simulink model "hcci_eng"  (R2018a)
settings: Solver=VariableStepAuto  StartTime=0.0  StopTime=t_end  RelTol=1e-3
values from neighbouring files (symbols this model uses):
  A01 = f(90)    [load_param.m]
  A2 = 0.3149    [load_param.m]
  A20 = f(70)    [load_param.m]
  alpha = 0.5794    [load_param.m]
  beta_0 = 1.035    [load_param.m]
  beta_1 = 1.1568    [load_param.m]
  gamma = 1.4    [load_param.m]
  h2 = 267    [load_param.m]
  kappa_0 = 0.5729    [load_param.m]
  kappa_1 = -0.52039    [load_param.m]
  m1_0 = states(end,1)    [hcci_sim.m]
  m2_0 = states(end,3)    [hcci_sim.m]
  p0 = 101000    [load_param.m]
  p2_0 = states(end,2)    [hcci_sim.m]
  R = 296.25    [HCCI_Combustion.m]    (also in load_param.m)
  T1 = 90 + 273.15    (= 363.15)    [load_param.m]
  T_w = 400    [load_param.m]
  tau = 120/N    (= 0.12)    [Validation.m]    (also in load_param.m)
  u_rbl = 3    [load_param.m]
  V1 = 0.0013    [load_param.m]
  V2 = 0.015    [load_param.m]
  V_BDC = V_ivc    (= 0.000592307692308)    [load_param.m]
  V_ivc = double(subs(Vc, theta, theta_ivc))    [HCCI_Combustion.m]    (also in load_param.m = 0.000592307692308)
  Wf = 11.9e-6    (= 1.19e-05)    [load_param.m]
undefined symbols (not defined in the file or in its folder): C_d
settings Model: Creator=Lenovo  LastModifiedBy=Lenovo

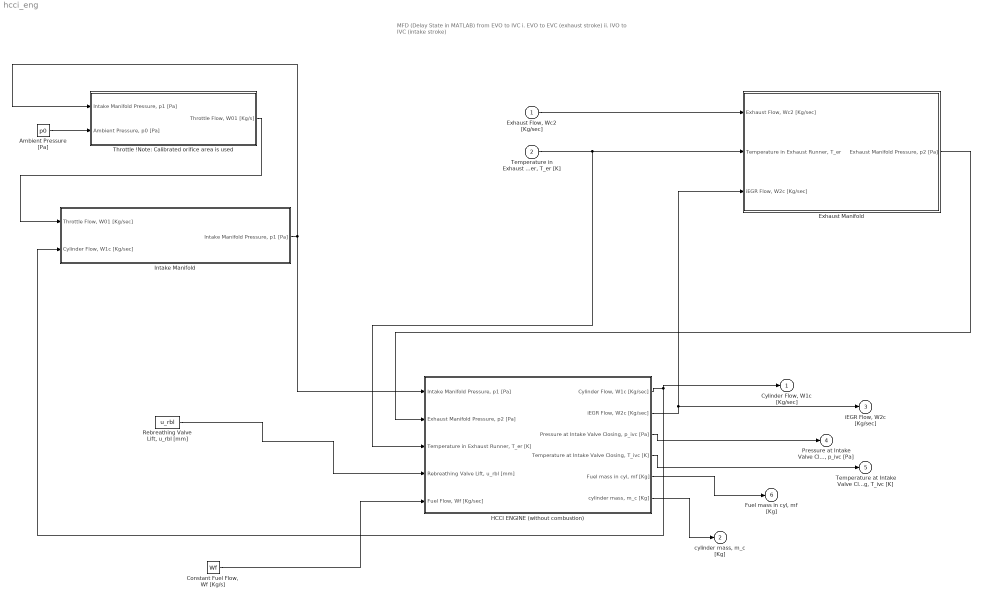
== system hcci_eng ==
  note: MFD (Delay State in MATLAB) from EVO to IVC
      | i. EVO to EVC (exhaust stroke)
      | ii. IVO to IVC (intake stroke)
  "Exhaust Flow, Wc2 [Kg/sec]" : Inport
  "Temperature in Exhaust Runner, T_er [K]" : Inport  Port=2
  Ambient Pressure [Pa] : Constant  Value=p0
  "Constant Fuel Flow, Wf [Kg/s] " : Constant  Value=Wf
  Exhaust Manifold : Subsystem
  HCCI ENGINE (without combustion) : Subsystem
  Intake Manifold : Subsystem
  "Rebreathing Valve Lift, u_rbl [mm]" : Constant  Value=u_rbl
  Throttle !Note: Calibrated orifice area is used : Subsystem
  "Cylinder Flow, W1c [Kg/sec]" : Outport
  "cylinder mass, m_c [Kg]" : Outport  Port=2
  "iEGR Flow, W2c [Kg/sec]" : Outport  Port=3
  "Pressure at Intake Valve Closing, p_ivc [Pa]" : Outport  Port=4
  "Temperature at Intake Valve Closing, T_ivc [K]" : Outport  Port=5
  "Fuel mass in cyl, mf [Kg]" : Outport  Port=6
  wires:
  Ambient Pressure [Pa]/1 -> Throttle !Note: Calibrated orifice area is used/2("Ambient Pressure, p0 [Pa]")
  Throttle !Note: Calibrated orifice area is used/1("Throttle Flow, W01 [Kg/s]") -> Intake Manifold/1("Throttle Flow, W01 [Kg/sec]")
  Intake Manifold/1("Intake Manifold Pressure, p1 [Pa]") -> HCCI ENGINE (without combustion)/1("Intake Manifold Pressure, p1 [Pa]"), Throttle !Note: Calibrated orifice area is used/1("Intake Manifold Pressure, p1 [Pa]")
  HCCI ENGINE (without combustion)/2("iEGR Flow, W2c [Kg/sec]") -> Exhaust Manifold/3("iEGR Flow, W2c [Kg/sec]"), "iEGR Flow, W2c [Kg/sec]"/1
  "Exhaust Flow, Wc2 [Kg/sec]"/1 -> Exhaust Manifold/1("Exhaust Flow, Wc2 [Kg/sec]")
  "Temperature in Exhaust Runner, T_er [K]"/1 -> Exhaust Manifold/2("Temperature in Exhaust Runner, T_er"), HCCI ENGINE (without combustion)/3("Temperature in Exhaust Runner, T_er [K]")
  Exhaust Manifold/1("Exhaust Manifold Pressure, p2 [Pa]") -> HCCI ENGINE (without combustion)/2("Exhaust Manifold Pressure, p2 [Pa]")
  "Constant Fuel Flow, Wf [Kg/s] "/1 -> HCCI ENGINE (without combustion)/5("Fuel Flow, Wf [Kg/sec] ")
  "Rebreathing Valve Lift, u_rbl [mm]"/1 -> HCCI ENGINE (without combustion)/4("Rebreathing Valve Lift, u_rbl [mm]")
  HCCI ENGINE (without combustion)/1("Cylinder Flow, W1c [Kg/sec]") -> "Cylinder Flow, W1c [Kg/sec]"/1, Intake Manifold/2("Cylinder Flow, W1c [Kg/sec]")
  HCCI ENGINE (without combustion)/3("Pressure at Intake Valve Closing, p_ivc [Pa]") -> "Pressure at Intake Valve Closing, p_ivc [Pa]"/1
  HCCI ENGINE (without combustion)/4("Temperature at Intake Valve Closing, T_ivc [K]") -> "Temperature at Intake Valve Closing, T_ivc [K]"/1
  HCCI ENGINE (without combustion)/5("Fuel mass in cyl, mf [Kg]") -> "Fuel mass in cyl, mf [Kg]"/1
  HCCI ENGINE (without combustion)/6("cylinder mass, m_c [Kg]") -> "cylinder mass, m_c [Kg]"/1

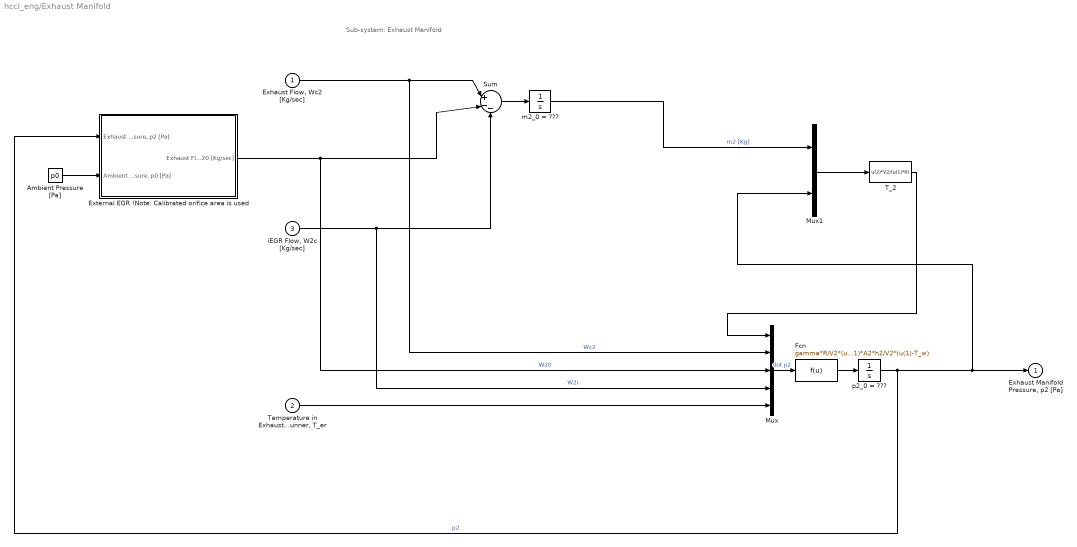
== system hcci_eng/Exhaust Manifold ==
  note: Sub-system: Exhaust Manifold
  "Exhaust Flow, Wc2 [Kg/sec]" : Inport
  "Temperature in Exhaust Runner, T_er" : Inport  Port=2
  "iEGR Flow, W2c [Kg/sec]" : Inport  Port=3
  Ambient Pressure [Pa] : Constant  Value=p0
  "External EGR !Note: Calibrated orifice area is used " : Subsystem
  Fcn : Fcn  Expr=gamma*R/V2*(u(2)*u(5)-(u(3)+u(4))*u(1))-(gamma-1)*A2*h2/V2*(u(1)-T_w)
  Mux : Mux  Inputs=5
  Mux1 : Mux  Inputs=2
  Sum : Sum  Inputs=|+--
  T_2 : Fcn  Expr=u(2)*V2/(u(1)*R)
  m2_0 = ??? : Integrator  InitialCondition=m2_0
  p2_0 = ??? : Integrator  InitialCondition=p2_0
  "Exhaust Manifold Pressure, p2 [Pa]" : Outport
  wires:
  "Exhaust Flow, Wc2 [Kg/sec]"/1 -> Mux/2, Sum/1  "Wc2"
  "External EGR !Note: Calibrated orifice area is used "/1("Exhaust Flow, W20 [Kg/sec]") -> Mux/3, Sum/2  "W20"
  "iEGR Flow, W2c [Kg/sec]"/1 -> Mux/4, Sum/3  "W2c"
  Sum/1 -> m2_0 = ???/1
  p2_0 = ???/1 -> Mux1/2, "Exhaust Manifold Pressure, p2 [Pa]"/1, "External EGR !Note: Calibrated orifice area is used "/1("Exhaust Manifold Pressure, p2 [Pa]")  "p2"
  Ambient Pressure [Pa]/1 -> "External EGR !Note: Calibrated orifice area is used "/2("Ambient Pressure, p0 [Pa]")
  "Temperature in Exhaust Runner, T_er"/1 -> Mux/5
  T_2/1 -> Mux/1
  Mux/1 -> Fcn/1  "dot p2"
  Fcn/1 -> p2_0 = ???/1
  Mux1/1 -> T_2/1
  m2_0 = ???/1 -> Mux1/1  "m2 [Kg]"

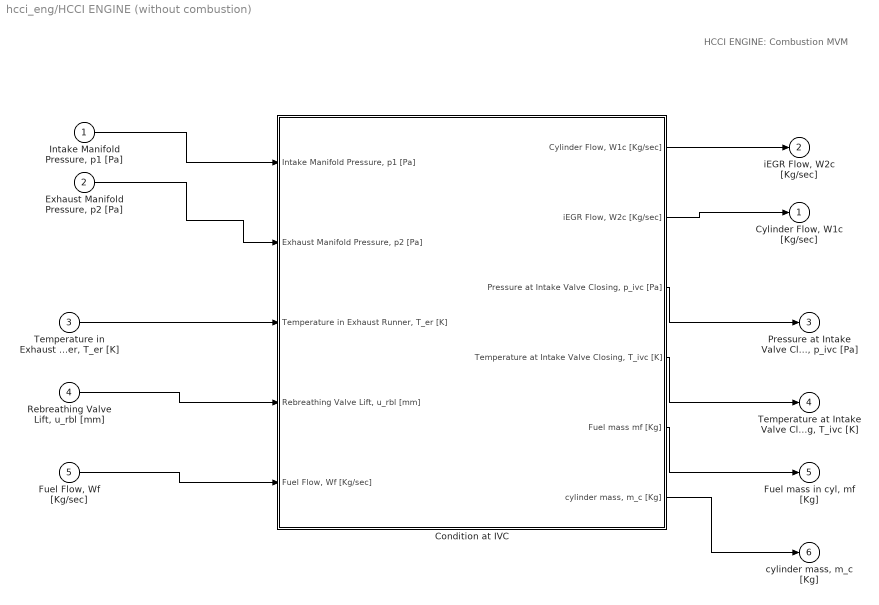
== system hcci_eng/HCCI ENGINE (without combustion) ==
  note: HCCI ENGINE: Combustion MVM
  "Intake Manifold Pressure, p1 [Pa]" : Inport
  "Exhaust Manifold Pressure, p2 [Pa]" : Inport  Port=2
  "Temperature in Exhaust Runner, T_er [K]" : Inport  Port=3
  "Rebreathing Valve Lift, u_rbl [mm]" : Inport  Port=4
  "Fuel Flow, Wf [Kg/sec] " : Inport  Port=5
  Condition at IVC : Subsystem
  "Cylinder Flow, W1c [Kg/sec]" : Outport
  "iEGR Flow, W2c [Kg/sec]" : Outport  Port=2
  "Pressure at Intake Valve Closing, p_ivc [Pa]" : Outport  Port=3
  "Temperature at Intake Valve Closing, T_ivc [K]" : Outport  Port=4
  "Fuel mass in cyl, mf [Kg]" : Outport  Port=5
  "cylinder mass, m_c [Kg]" : Outport  Port=6
  wires:
  "Intake Manifold Pressure, p1 [Pa]"/1 -> Condition at IVC/1("Intake Manifold Pressure, p1 [Pa]")
  "Exhaust Manifold Pressure, p2 [Pa]"/1 -> Condition at IVC/2("Exhaust Manifold Pressure, p2 [Pa]")
  "Temperature in Exhaust Runner, T_er [K]"/1 -> Condition at IVC/3("Temperature in Exhaust Runner, T_er [K]")
  "Rebreathing Valve Lift, u_rbl [mm]"/1 -> Condition at IVC/4("Rebreathing Valve Lift, u_rbl [mm]")
  "Fuel Flow, Wf [Kg/sec] "/1 -> Condition at IVC/5("Fuel Flow, Wf [Kg/sec] ")
  Condition at IVC/1("Cylinder Flow, W1c [Kg/sec]") -> "iEGR Flow, W2c [Kg/sec]"/1
  Condition at IVC/2("iEGR Flow, W2c [Kg/sec]") -> "Cylinder Flow, W1c [Kg/sec]"/1
  Condition at IVC/3("Pressure at Intake Valve Closing, p_ivc [Pa]") -> "Pressure at Intake Valve Closing, p_ivc [Pa]"/1
  Condition at IVC/4("Temperature at Intake Valve Closing, T_ivc [K]") -> "Temperature at Intake Valve Closing, T_ivc [K]"/1
  Condition at IVC/5(Fuel mass mf [Kg]) -> "Fuel mass in cyl, mf [Kg]"/1
  Condition at IVC/6("cylinder mass, m_c [Kg]") -> "cylinder mass, m_c [Kg]"/1

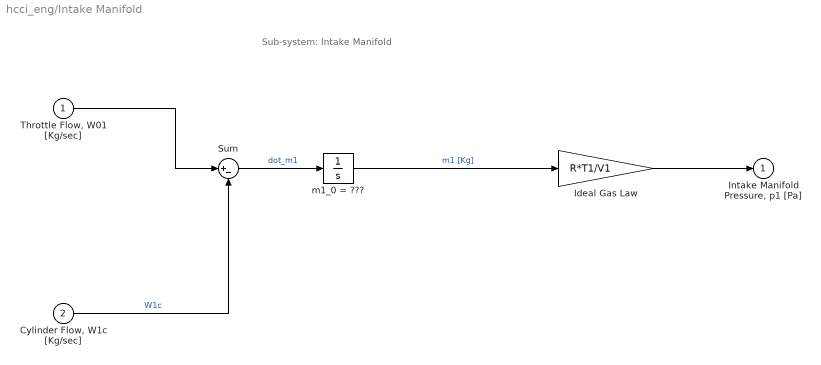
== system hcci_eng/Intake Manifold ==
  note: Sub-system: Intake Manifold
  "Throttle Flow, W01 [Kg/sec]" : Inport
  "Cylinder Flow, W1c [Kg/sec]" : Inport  Port=2
  Ideal Gas Law : Gain  Gain=R*T1/V1
  Sum : Sum  Inputs=|+-
  m1_0 = ??? : Integrator  InitialCondition=m1_0
  "Intake Manifold Pressure, p1 [Pa]" : Outport
  wires:
  "Cylinder Flow, W1c [Kg/sec]"/1 -> Sum/2  "W1c"
  "Throttle Flow, W01 [Kg/sec]"/1 -> Sum/1
  Sum/1 -> m1_0 = ???/1  "dot_m1"
  m1_0 = ???/1 -> Ideal Gas Law/1  "m1 [Kg]"
  Ideal Gas Law/1 -> "Intake Manifold Pressure, p1 [Pa]"/1

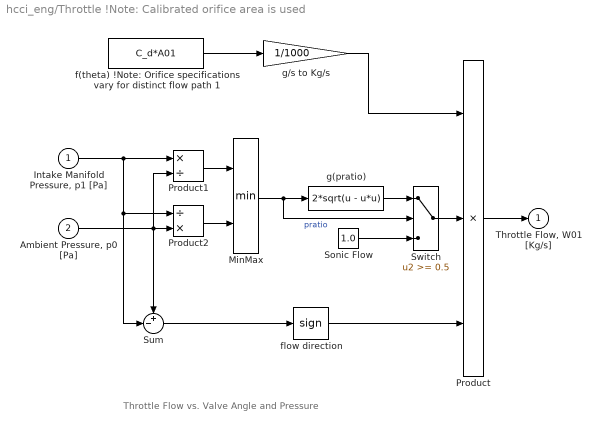
== system hcci_eng/Throttle !Note: Calibrated orifice area is used ==
  note: Throttle Flow vs. Valve Angle and Pressure
  "Intake Manifold Pressure, p1 [Pa]" : Inport
  "Ambient Pressure, p0 [Pa]" : Inport  Port=2
  MinMax : MinMax  Inputs=2  SaturateOnIntegerOverflow=on  InputSameDT=on
  Product : Product  Inputs=3  SaturateOnIntegerOverflow=on  RndMeth=Zero  InputSameDT=on  OutDataTypeStr=Inherit: Same as first input
  Product1 : Product  Inputs=*/  SaturateOnIntegerOverflow=on  RndMeth=Zero  InputSameDT=on  OutDataTypeStr=Inherit: Same as first input
  Product2 : Product  Inputs=/*  SaturateOnIntegerOverflow=on  RndMeth=Zero  InputSameDT=on  OutDataTypeStr=Inherit: Same as first input
  "Sonic Flow " : Constant  Value=1.0
  Sum : Sum  Inputs=+-|  SaturateOnIntegerOverflow=on  InputSameDT=on  OutDataTypeStr=Inherit: Same as first input
  Switch : Switch  Threshold=0.5  SaturateOnIntegerOverflow=on  InputSameDT=on
  f(theta) !Note: Orifice specifications vary for distinct flow path 1 : Constant  Value=C_d*A01
  flow direction : Signum
  g(pratio) : Fcn  Expr=2*sqrt(u - u*u)
  g/s to Kg/s : Gain  Gain=1/1000
  "Throttle Flow, W01 [Kg/s]" : Outport  InitialOutput=0
  wires:
  "Intake Manifold Pressure, p1 [Pa]"/1 -> Sum/2, Product2/1, Product1/1
  Product2/1 -> MinMax/2
  Product1/1 -> MinMax/1
  "Ambient Pressure, p0 [Pa]"/1 -> Sum/1, Product2/2, Product1/2
  g(pratio)/1 -> Switch/1
  "Sonic Flow "/1 -> Switch/3
  Switch/1 -> Product/2
  flow direction/1 -> Product/3
  Sum/1 -> flow direction/1
  MinMax/1 -> Switch/2, g(pratio)/1  "pratio"
  Product/1 -> "Throttle Flow, W01 [Kg/s]"/1
  f(theta) !Note: Orifice specifications vary for distinct flow path 1/1 -> g/s to Kg/s/1
  g/s to Kg/s/1 -> Product/1

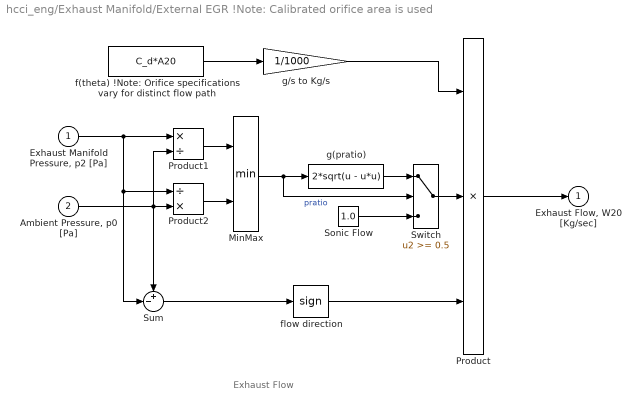
== system hcci_eng/Exhaust Manifold/External EGR !Note: Calibrated orifice area is used  ==
  note: Exhaust Flow
  "Exhaust Manifold Pressure, p2 [Pa]" : Inport
  "Ambient Pressure, p0 [Pa]" : Inport  Port=2
  MinMax : MinMax  Inputs=2  SaturateOnIntegerOverflow=on  InputSameDT=on
  Product : Product  Inputs=3  SaturateOnIntegerOverflow=on  RndMeth=Zero  InputSameDT=on  OutDataTypeStr=Inherit: Same as first input
  Product1 : Product  Inputs=*/  SaturateOnIntegerOverflow=on  RndMeth=Zero  InputSameDT=on  OutDataTypeStr=Inherit: Same as first input
  Product2 : Product  Inputs=/*  SaturateOnIntegerOverflow=on  RndMeth=Zero  InputSameDT=on  OutDataTypeStr=Inherit: Same as first input
  "Sonic Flow " : Constant  Value=1.0
  Sum : Sum  Inputs=+-|  SaturateOnIntegerOverflow=on  InputSameDT=on  OutDataTypeStr=Inherit: Same as first input
  Switch : Switch  Threshold=0.5  SaturateOnIntegerOverflow=on  InputSameDT=on
  "f(theta) !Note: Orifice specifications vary for distinct flow path " : Constant  Value=C_d*A20
  flow direction : Signum
  g(pratio) : Fcn  Expr=2*sqrt(u - u*u)
  g/s to Kg/s : Gain  Gain=1/1000
  "Exhaust Flow, W20 [Kg/sec]" : Outport  InitialOutput=0
  wires:
  "Exhaust Manifold Pressure, p2 [Pa]"/1 -> Sum/2, Product2/1, Product1/1
  Product2/1 -> MinMax/2
  Product1/1 -> MinMax/1
  "Ambient Pressure, p0 [Pa]"/1 -> Sum/1, Product2/2, Product1/2
  g(pratio)/1 -> Switch/1
  "Sonic Flow "/1 -> Switch/3
  Switch/1 -> Product/2
  flow direction/1 -> Product/3
  Sum/1 -> flow direction/1
  MinMax/1 -> Switch/2, g(pratio)/1  "pratio"
  Product/1 -> "Exhaust Flow, W20 [Kg/sec]"/1
  "f(theta) !Note: Orifice specifications vary for distinct flow path "/1 -> g/s to Kg/s/1
  g/s to Kg/s/1 -> Product/1

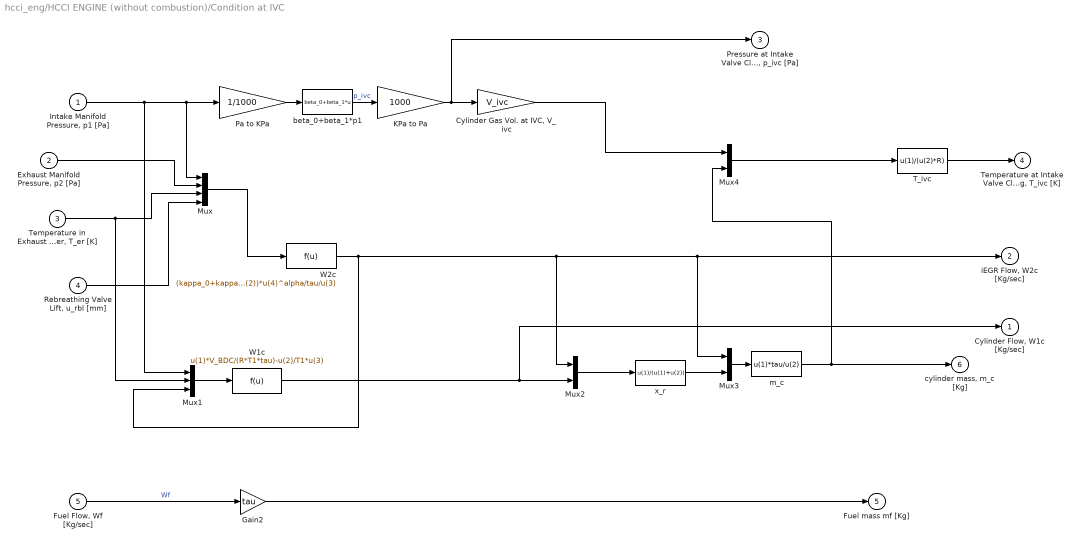
== system hcci_eng/HCCI ENGINE (without combustion)/Condition at IVC ==
  "Intake Manifold Pressure, p1 [Pa]" : Inport
  "Exhaust Manifold Pressure, p2 [Pa]" : Inport  Port=2
  "Temperature in Exhaust Runner, T_er [K]" : Inport  Port=3
  "Rebreathing Valve Lift, u_rbl [mm]" : Inport  Port=4
  "Fuel Flow, Wf [Kg/sec] " : Inport  Port=5
  "Cylinder Gas Vol. at IVC, V_ivc" : Gain  Gain=V_ivc
  Gain2 : Gain  Gain=tau
  KPa to Pa : Gain  Gain=1000
  Mux : Mux
  Mux1 : Mux  Inputs=3
  Mux2 : Mux  Inputs=2
  Mux3 : Mux  Inputs=2
  Mux4 : Mux  Inputs=2
  Pa to KPa : Gain  Gain=1/1000
  T_ivc : Fcn  Expr=u(1)/(u(2)*R)
  W1c : Fcn  Expr=u(1)*V_BDC/(R*T1*tau)-u(2)/T1*u(3)
  W2c : Fcn  Expr=(kappa_0+kappa_1*u(1)/u(2))*u(4)^alpha/tau/u(3)
  beta_0+beta_1*p1 : Fcn  Expr=beta_0+beta_1*u
  m_c : Fcn  Expr=u(1)*tau/u(2)
  x_r : Fcn  Expr=u(1)/(u(1)+u(2))
  "Cylinder Flow, W1c [Kg/sec]" : Outport
  "iEGR Flow, W2c [Kg/sec]" : Outport  Port=2
  "Pressure at Intake Valve Closing, p_ivc [Pa]" : Outport  Port=3
  "Temperature at Intake Valve Closing, T_ivc [K]" : Outport  Port=4
  Fuel mass mf [Kg] : Outport  Port=5
  "cylinder mass, m_c [Kg]" : Outport  Port=6
  wires:
  beta_0+beta_1*p1/1 -> KPa to Pa/1  "p_ivc"
  Mux/1 -> W2c/1
  "Temperature in Exhaust Runner, T_er [K]"/1 -> Mux1/2, Mux/3
  "Rebreathing Valve Lift, u_rbl [mm]"/1 -> Mux/4
  "Fuel Flow, Wf [Kg/sec] "/1 -> Gain2/1  "Wf"
  "Intake Manifold Pressure, p1 [Pa]"/1 -> Mux1/1, Mux/1, Pa to KPa/1
  "Exhaust Manifold Pressure, p2 [Pa]"/1 -> Mux/2
  Pa to KPa/1 -> beta_0+beta_1*p1/1
  KPa to Pa/1 -> "Pressure at Intake Valve Closing, p_ivc [Pa]"/1, "Cylinder Gas Vol. at IVC, V_ivc"/1
  Gain2/1 -> Fuel mass mf [Kg]/1
  Mux1/1 -> W1c/1
  W2c/1 -> Mux1/3, Mux3/1, "iEGR Flow, W2c [Kg/sec]"/1, Mux2/1
  W1c/1 -> Mux2/2, "Cylinder Flow, W1c [Kg/sec]"/1
  Mux2/1 -> x_r/1
  Mux3/1 -> m_c/1
  x_r/1 -> Mux3/2
  m_c/1 -> Mux4/2, "cylinder mass, m_c [Kg]"/1
  "Cylinder Gas Vol. at IVC, V_ivc"/1 -> Mux4/1
  Mux4/1 -> T_ivc/1
  T_ivc/1 -> "Temperature at Intake Valve Closing, T_ivc [K]"/1
